simulink model "Navigation_KF_Subsystem_child"  (R2016a)
settings: configuration reference "AR_Drone_ConfigSet" (kept outside this file)
undefined symbols (not defined in the file or in its folder): Accel_Calib_Gain, Accel_Calib_Offset, DiscIntNeverNeededParam, Mag_Calib_Gain_Vector, Mag_Calib_Offset_Vector
libraries: aerolibtransform2 x4, vrlib x4
(part 2 of 2)

== matlab function Navigation_KF_Subsystem_child/Kalman Filter/Re-Align Yaw Axis ==
  data: DroneStatus input; ResetTrigger output; initial_condition output
function [ResetTrigger,initial_condition]= fcn(DroneStatus)
%#codegen


if (DroneStatus == Drone_StateModeType.Landing_Terminate || DroneStatus == Drone_StateModeType.WaitForHost || DroneStatus == Drone_StateModeType.Initialize) %MotorArmed = 0
    ResetTrigger = 1;
else
    ResetTrigger = 0;  %enable for Controlled_Flight and Landing_Sequence
end                    %MotorArmed = 1 in this state

initial_condition = 0;

== matlab function Navigation_KF_Subsystem_child/Sensor Fusion1/Magnetometer Processing/Magnetometer Heading Calculation/Compensate for Magnetic Declination (~60 degrees in Boston)_ ==
  data: vector_in input; y output
function y = fcn(vector_in)
%#codegen

% %  WHY WAS THIS COMMENTED OUT???
% %  Reason: While the intention to rotate 60 degrees up north was in good
% %  intention, the math was not correct: you are rotating in the global
% %  reference frame, an axis which stays fixed. we want to rotate upwards
% %  along an axis which is perpindicular to the XY coordinates
% %

%transform the pitch up, recall that in SL3D the x-axis = z-axis
%                                                y-axis = x-axis

rotation = 1*pi/3;
C_term = cos(rotation);
S_term = sin(rotation);
MatrixY = [C_term 0 -S_term; 0 1 0; S_term 0 C_term ];
MatrixX = [1 0 0; 0 C_term -S_term; 0 S_term C_term ];


y = MatrixY*vector_in;

== matlab function Navigation_KF_Subsystem_child/Sensor Fusion1/Magnetometer Processing/Magnetometer Heading Calculation/Compensate for Magnetic Declination (~67 degrees in Boston)_2 ==
  data: vector_in input; y output; declination_ang input
function y = fcn(vector_in, declination_ang)

B_xy = norm([vector_in(1) vector_in(2)]);
B_z = vector_in(3);

Declination_Angle = -atan2(B_z,B_xy);


% Declination_Angle = declination_ang*pi/180;

rot_axis = [vector_in(2) -vector_in(1)]; %find a vector perpindicular to the XY vector, such that we can pitch around it
rot_axis = rot_axis/norm(rot_axis);
%rotate by this amount
% for i=1:1:45;
% rot_angle = i*(pi/180) ;

%Define new rotation matrix
C_term = cos(Declination_Angle);
S_term = sin(Declination_Angle);
t = 1-C_term;
ux = rot_axis(1);
uy = rot_axis(2);
uz = 0; 

new_rot = [(t*ux^2 + C_term) (t*ux*uy-S_term*uz) (t*ux*uz+S_term*uy)
           (t*ux*uy+S_term*uz) (t*uy^2+C_term)     (t*uy*uz - S_term*ux)
           (t*ux*uz - S_term*uy) (t*uy*uz+S_term*ux) (t*uz^2 + C_term)];


y = new_rot*vector_in;

== matlab function Navigation_KF_Subsystem_child/Sensor Fusion1/Re-Align Yaw Axis ==
  data: DroneStatus input; ResetTrigger output; initial_condition output
function [ResetTrigger,initial_condition]= fcn(DroneStatus)
%#codegen


if (DroneStatus == Drone_StateModeType.Landing_Terminate || DroneStatus == Drone_StateModeType.WaitForHost || DroneStatus == Drone_StateModeType.Initialize) %MotorArmed = 0
    ResetTrigger = 1;
else
    ResetTrigger = 0;  %enable for Controlled_Flight and Landing_Sequence
end                    %MotorArmed = 1 in this state

initial_condition = 0;

== matlab function Navigation_KF_Subsystem_child/Sensor Fusion1/Ultrasound Estimator/Kalman Tracker ==
  data: UltraSoundMeasure input; state_correction output; covariance_correction output; covariance_correction_input input; state_correction_input input
function [state_correction, covariance_correction] = fcn(UltraSoundMeasure, covariance_correction_input,state_correction_input)


%-------------------------------
%-------------------------------
%---- Predict Stage ------------
%-------------------------------
%-------------------------------

%our states:
%  [Wx Wy Wz Bx By Bz   ]
%

p_var = 1e-2;
Ts = 1/400;
%Process Noise

Q = [p_var^2     0     
      0         p_var^2 ];

%A matrix
A =  [1   Ts    
      0   1];

%odutput these values with a unit delay (for algebraic loop), apply initial conditions
state_prediction = A*state_correction_input;
covariance_prediction_ = A*covariance_correction_input*A' + Q;

%-------------------------------
%-------------------------------
%---- Estimate Stage -----------
%-------------------------------
%-------------------------------
    %H matrix
    H = [1 0];

    %Measurement noise
    m_var = 1;
%     m_var_r = 1;

    R = [m_var^2];

    %Measurement Z
    Z = UltraSoundMeasure;

    %Compute Kalman Gain
    Kalman_Gain = covariance_prediction_*H'*inv(H*covariance_prediction_*H'+R); %2x2 matrix

    %compute state space correction based on measurement
    state_correction = state_prediction + Kalman_Gain*(Z - H*state_prediction); %2x1 vector of states

    %compute covariance correction
    covariance_correction = (eye(2) - Kalman_Gain*H)*covariance_prediction_; %2x2 covariance matrix

end

== matlab function Navigation_KF_Subsystem_child/Kalman Filter/KF_ROLL/Kalman Tracker ==
  data: prev_state input; covariance_correction_prev input; state_correction output; covariance_correction output; ctrl_input_gyro input; measurement_angle input
function [state_correction, covariance_correction] = fcn(prev_state, covariance_correction_prev, ctrl_input_gyro, measurement_angle)


%-------------------------------
%-------------------------------
%---- Predict Stage ------------
%-------------------------------
%-------------------------------
% pix_value = 5;
Ts = 1/400;
%Process Noise
p_var =0.01;
Q = [p_var^2     0         
      0         p_var^2];

%A matrix
A =  [1   -Ts 
      0   1];

%odutput these values with a unit delay (for algebraic loop), apply initial conditions
state_prediction = A*prev_state + [Ts 0; 0 0]*[ctrl_input_gyro; 0 ];
covariance_prediction = A*covariance_correction_prev*A' + Q;

%-------------------------------
%-------------------------------
%---- Estimate Stage -----------
%-------------------------------
%-------------------------------

    %H matrix
    H = [1 0];

    %Measurement noise from accelerometer angle measurement
    m_var = 0.5;
%     m_var_r = 1;

    R = [m_var^2 ];

    %Measurement Z
    Z = [measurement_angle];

    %Compute Kalman Gain
    Kalman_Gain = covariance_prediction*H'*inv(H*covariance_prediction*H'+R); %2x2 matrix

    %compute state space correction based on measurement
    state_correction = state_prediction + Kalman_Gain*(Z - H*state_prediction); %4x1 vector of states

    %compute covariance correction
    covariance_correction = (eye(2) - Kalman_Gain*H)*covariance_prediction; %2x2 covariance matrix

%     corrected_angle_measure = state_correction(1) - Ts*state_correction(2);
end

== matlab function Navigation_KF_Subsystem_child/Kalman Filter/KF_PITCH/Kalman Tracker ==
  data: prev_state input; covariance_correction_prev input; state_correction output; covariance_correction output; ctrl_input_gyro input; measurement_angle input
function [state_correction, covariance_correction] = fcn(prev_state, covariance_correction_prev, ctrl_input_gyro, measurement_angle)


%-------------------------------
%-------------------------------
%---- Predict Stage ------------
%-------------------------------
%-------------------------------
% pix_value = 5;
Ts = 1/400;
%Process Noise
p_var =0.01;
Q = [p_var^2     0         
      0         p_var^2];

%A matrix
A =  [1   -Ts 
      0   1];

%odutput these values with a unit delay (for algebraic loop), apply initial conditions
state_prediction = A*prev_state + [Ts 0; 0 0]*[ctrl_input_gyro; 0 ];
covariance_prediction = A*covariance_correction_prev*A' + Q;

%-------------------------------
%-------------------------------
%---- Estimate Stage -----------
%-------------------------------
%-------------------------------

    %H matrix
    H = [1 0];

    %Measurement noise from accelerometer angle measurement
    m_var = 1;
%     m_var_r = 1;

    R = [m_var^2 ];

    %Measurement Z
    Z = [measurement_angle];

    %Compute Kalman Gain
    Kalman_Gain = covariance_prediction*H'*inv(H*covariance_prediction*H'+R); %2x2 matrix

    %compute state space correction based on measurement
    state_correction = state_prediction + Kalman_Gain*(Z - H*state_prediction); %4x1 vector of states

    %compute covariance correction
    covariance_correction = (eye(2) - Kalman_Gain*H)*covariance_prediction; %2x2 covariance matrix

%     corrected_angle_measure = state_correction(1) - Ts*state_correction(2);
end

== matlab function Navigation_KF_Subsystem_child/Kalman Filter/Ultrasound Estimator/Kalman Tracker ==
  data: UltraSoundMeasure input; state_correction output; covariance_correction output; covariance_correction_input input; state_correction_input input
function [state_correction, covariance_correction] = fcn(UltraSoundMeasure, covariance_correction_input,state_correction_input)


%-------------------------------
%-------------------------------
%---- Predict Stage ------------
%-------------------------------
%-------------------------------

%our states:
%  [Wx Wy Wz Bx By Bz   ]
%

p_var = 1e-2;
Ts = 1/400;
%Process Noise

Q = [p_var^2     0     
      0         p_var^2 ];

%A matrix
A =  [1   Ts    
      0   1];

%odutput these values with a unit delay (for algebraic loop), apply initial conditions
state_prediction = A*state_correction_input;
covariance_prediction_ = A*covariance_correction_input*A' + Q;

%-------------------------------
%-------------------------------
%---- Estimate Stage -----------
%-------------------------------
%-------------------------------
    %H matrix
    H = [1 0];

    %Measurement noise
    m_var = 1;
%     m_var_r = 1;

    R = [m_var^2];

    %Measurement Z
    Z = UltraSoundMeasure;

    %Compute Kalman Gain
    Kalman_Gain = covariance_prediction_*H'*inv(H*covariance_prediction_*H'+R); %2x2 matrix

    %compute state space correction based on measurement
    state_correction = state_prediction + Kalman_Gain*(Z - H*state_prediction); %2x1 vector of states

    %compute covariance correction
    covariance_correction = (eye(2) - Kalman_Gain*H)*covariance_prediction_; %2x2 covariance matrix

end

== matlab function Navigation_KF_Subsystem_child/Kalman Filter/VRML_Calculations/Magnetometer Heading Calculation/Compensate for Magnetic Declination (~60 degrees in Boston)_ ==
  data: vector_in input; y output
function y = fcn(vector_in)
%#codegen

% %  WHY WAS THIS COMMENTED OUT???
% %  Reason: While the intention to rotate 60 degrees up north was in good
% %  intention, the math was not correct: you are rotating in the global
% %  reference frame, an axis which stays fixed. we want to rotate upwards
% %  along an axis which is perpindicular to the XY coordinates
% %

%transform the pitch up, recall that in SL3D the x-axis = z-axis
%                                                y-axis = x-axis

rotation = 1*pi/3;
C_term = cos(rotation);
S_term = sin(rotation);
MatrixY = [C_term 0 -S_term; 0 1 0; S_term 0 C_term ];
MatrixX = [1 0 0; 0 C_term -S_term; 0 S_term C_term ];


y = MatrixY*vector_in;

== matlab function Navigation_KF_Subsystem_child/Kalman Filter/VRML_Calculations/Magnetometer Heading Calculation/Compensate for Magnetic Declination (~67 degrees in Boston)_2 ==
  data: vector_in input; y output; declination_ang input
function y = fcn(vector_in, declination_ang)

B_xy = norm([vector_in(1) vector_in(2)]);
B_z = vector_in(3);

Declination_Angle = -atan2(B_z,B_xy);


% Declination_Angle = declination_ang*pi/180;

rot_axis = [vector_in(2) -vector_in(1)]; %find a vector perpindicular to the XY vector, such that we can pitch around it
rot_axis = rot_axis/norm(rot_axis);
%rotate by this amount
% for i=1:1:45;
% rot_angle = i*(pi/180) ;

%Define new rotation matrix
C_term = cos(Declination_Angle);
S_term = sin(Declination_Angle);
t = 1-C_term;
ux = rot_axis(1);
uy = rot_axis(2);
uz = 0; 

new_rot = [(t*ux^2 + C_term) (t*ux*uy-S_term*uz) (t*ux*uz+S_term*uy)
           (t*ux*uy+S_term*uz) (t*uy^2+C_term)     (t*uy*uz - S_term*ux)
           (t*ux*uz - S_term*uy) (t*uy*uz+S_term*ux) (t*uz^2 + C_term)];


y = new_rot*vector_in;
